simulink model "VINS"  (R2018a)
settings: Solver=FixedStepDiscrete  StartTime=0.0  StopTime=inf  FixedStep=1/Fs  RelTol=1e-3  EnableMultiTasking=on
PreLoadFcn:
  | modelDef = getModelDef(calibrateSFMA);
  | 
  | %imuPar = getImuPar('lmvpUncalibrated');
  | 
  | timeMatchThreshold = 1000;
undefined symbols (not defined in the file or in its folder): beep, dejitter_on, Fs, homogeneous3x4Transform_k_kmin1, imuLocationMm, imuPar, numStates, simData, tstamp_k_us, tstamp_kmin1_us
libraries: simulink x69, dspmtrx3 x35, dspindex x9, vrlib x7, dspstat3 x7, dspinverses x6, dspsigops x5, dspmathops x2, rtwdemowidgets x1, dspfactors x1, simulink_extras x1
(part 1 of 6)
settings Model: SimulationMode=external  TunableVars=dejitter_on,imuLocationMm,imuPar  TunableVarsStorageClass=ExportedGlobal,ExportedGlobal,ExportedGlobal  TunableVarsTypeQualifier=,,const  Creator=Eric  LastModifiedBy=efoxlin
settings SolverCC: PositivePriorityOrder=on
settings DataIOCC: SaveOutput=off  SaveTime=off
settings OptimizationCC: DefaultParameterBehavior=Inlined  UseFloatMulNetSlope=on  DefaultUnderspecifiedDataType=single  UseSpecifiedMinMax=on  PassReuseOutputArgsAs=Individual arguments  NoFixptDivByZeroProtection=on  EfficientFloat2IntCast=on  LifeSpan=1  MaxStackSize=1000000  OptimizeBlockOrder=speed  DifferentSizesBufferReuse=on
settings DebuggingCC: ReadBeforeWriteMsg=DisableAll  WriteAfterWriteMsg=DisableAll  WriteAfterReadMsg=DisableAll  ParameterPrecisionLossMsg=none  ParameterTunabilityLossMsg=error  UnconnectedOutputMsg=none
settings HardwareCC: ProdBitPerPointer=32  ProdBitPerSizeT=32  ProdBitPerPtrDiffT=32  ProdLargestAtomicInteger=Long  ProdLargestAtomicFloat=Double  ProdWordSize=32  ProdHWDeviceType=ARM Compatible->ARM Cortex
settings SFSimCC: MATLABDynamicMemAlloc=off
settings RTWCC: SystemTargetFile=ert.tlc  GenCodeOnly=on  PackageGeneratedCodeAndArtifacts=on  TemplateMakefile=ert_default_tmf  GenerateReport=on  Toolchain=Linaro Toolchain v4.8  BuildConfiguration=Faster Runs  IncludeHyperlinkInReport=on  LaunchReport=on  PortableWordSizes=on  TargetLang=C++  GenerateTraceInfo=on  GenerateTraceReport=on  GenerateTraceReportSl=on  GenerateTraceReportSf=on  GenerateTraceReportEml=on  GenerateCodeReplacementReport=on
settings CodeAppCC: ForceParamTrailComments=on  IgnoreCustomStorageClasses=off  OperatorAnnotations=on  SimulinkDataObjDesc=on  SFDataObjDesc=on  InsertBlockDesc=on
settings ERTTargetCC: TargetLangStandard=C++03 (ISO)  CombineSignalStateStructs=on  SuppressErrorStatus=on  SupportAbsoluteTime=off  MultiInstanceERTCode=on  CodeInterfacePackaging=C++ class  SupportNonFinite=off  SupportComplex=off  SupportVariableSizeSignals=on  RootIOFormat=Structure reference  ERTCustomFileTemplate=example_file_process.tlc  ERTFilePackagingFormat=Compact

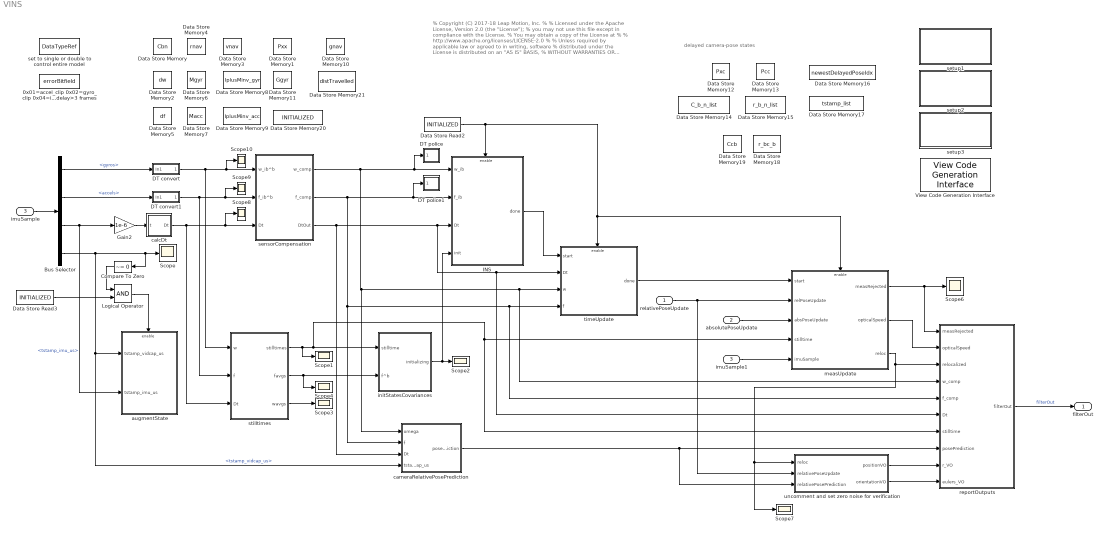
== system VINS ==
  note: delayed camera-pose states
  note: % Copyright (C) 2017-18 Leap Motion, Inc.
      | %
      | %    Licensed under the Apache License, Version 2.0 (the "License");
      | %    you may not use this file except in compliance with the License.
      | %    You may obtain a copy of the License at
      | %
      | %        http://www.apache.org/licenses/LICENSE-2.0
      | %
      | %    Unless required by applicable law or agreed to in writing, software
      | %    distributed under the License is distributed on an "AS IS" BASIS,
      | %    WITHOUT WARRANTIES OR CONDITIONS OF ANY KIND, either express or implied.
      | %    See the License for the specific language governing permissions and
      | %    limitations under the License.
      | % Author: Eric Foxlin
  relativePoseUpdate : Inport  OutDataTypeStr=Bus: relativePoseUpdate
  absolutePoseUpdate : Inport  Port=2  OutDataTypeStr=Bus: absolutePoseUpdate
  imuSample : Inport  Port=3  OutDataTypeStr=Bus: imuSample  PortDimensions=1
  0x01=accel_clip 0x02=gyro_clip 0x04=imu_dropout(>5ms) 0x08=vid_delay>3 frames : DataStoreMemory  DataStoreName=errorBitfield  ReadBeforeWriteMsg=warning  WriteAfterWriteMsg=warning  WriteAfterReadMsg=warning  InitialValue=uint32(0)  ShowAdditionalParam=off  OutDataTypeStr=uint32
  Bus Selector : BusSelector  OutputSignals=gyros,accels,tstamp_imu_us,tstamp_vidcap_us
  Compare To Zero : simulink/Logic and Bit Operations/Compare To Zero  relop=~=  OutDataTypeStr=boolean
  DT convert : Subsystem
  DT convert1 : Subsystem
  DT police : Subsystem  TreatAsAtomicUnit=on
  DT police1 : Subsystem  TreatAsAtomicUnit=on
  Data Store Memory : DataStoreMemory  DataStoreName=Cbn  ReadBeforeWriteMsg=warning  WriteAfterWriteMsg=warning  WriteAfterReadMsg=warning  InitialValue=eye(3)  VectorParams1D=off  ShowAdditionalParam=off
  Data Store Memory1 : DataStoreMemory  DataStoreName=Pxx  ReadBeforeWriteMsg=warning  WriteAfterWriteMsg=warning  WriteAfterReadMsg=warning  InitialValue=eye(modelDef.numStates)*1e-12  ShowAdditionalParam=off
  Data Store Memory10 : DataStoreMemory  DataStoreName=gnav  ReadBeforeWriteMsg=warning  WriteAfterWriteMsg=warning  WriteAfterReadMsg=warning  InitialValue=[0;0; 9.80665]  VectorParams1D=off  ShowAdditionalParam=off
  Data Store Memory11 : DataStoreMemory  DataStoreName=Ggyr  ReadBeforeWriteMsg=warning  WriteAfterWriteMsg=warning  WriteAfterReadMsg=warning  InitialValue=zeros(3,3)  VectorParams1D=off  ShowAdditionalParam=off
  Data Store Memory12 : DataStoreMemory  DataStoreName=Pxc  ReadBeforeWriteMsg=warning  WriteAfterWriteMsg=warning  WriteAfterReadMsg=warning  InitialValue=zeros(modelDef.numStates, modelDef.maxNumDelayedPoses * modelDef.statesPerDelayedPose)  ShowAdditionalParam=off
  Data Store Memory13 : DataStoreMemory  DataStoreName=Pcc  ReadBeforeWriteMsg=warning  WriteAfterWriteMsg=warning  WriteAfterReadMsg=warning  InitialValue=zeros(modelDef.statesPerDelayedPose*modelDef.maxNumDelayedPoses , modelDef.statesPerDelayedPose*modelDef.maxNumDelayedPoses )  ShowAdditionalParam=off
  Data Store Memory14 : DataStoreMemory  DataStoreName=C_b_n_list  ReadBeforeWriteMsg=warning  WriteAfterWriteMsg=warning  WriteAfterReadMsg=warning  InitialValue=zeros(3, 3, max(2,modelDef.maxNumDelayedPoses))  VectorParams1D=off  ShowAdditionalParam=off
  Data Store Memory15 : DataStoreMemory  DataStoreName=r_b_n_list  ReadBeforeWriteMsg=warning  WriteAfterWriteMsg=warning  WriteAfterReadMsg=warning  InitialValue=zeros(3, 1, max(2,modelDef.maxNumDelayedPoses))  VectorParams1D=off  ShowAdditionalParam=off
  Data Store Memory16 : DataStoreMemory  DataStoreName=newestDelayedPoseIdx  ReadBeforeWriteMsg=warning  WriteAfterWriteMsg=warning  WriteAfterReadMsg=warning  ShowAdditionalParam=off  OutDataTypeStr=uint8
  Data Store Memory17 : DataStoreMemory  DataStoreName=tstamp_list  ReadBeforeWriteMsg=warning  WriteAfterWriteMsg=warning  WriteAfterReadMsg=warning  InitialValue=zeros(modelDef.maxNumDelayedPoses, 1)  ShowAdditionalParam=off
  Data Store Memory18 : DataStoreMemory  DataStoreName=r_bc_b  ReadBeforeWriteMsg=warning  WriteAfterWriteMsg=warning  WriteAfterReadMsg=warning  InitialValue=-[-17.48; -4.5; 2.539]/1000  VectorParams1D=off  ShowAdditionalParam=off
  Data Store Memory19 : DataStoreMemory  DataStoreName=Ccb  ReadBeforeWriteMsg=warning  WriteAfterWriteMsg=warning  WriteAfterReadMsg=warning  InitialValue=eye(3)  VectorParams1D=off  ShowAdditionalParam=off
  Data Store Memory2 : DataStoreMemory  DataStoreName=dw  ReadBeforeWriteMsg=warning  WriteAfterWriteMsg=warning  WriteAfterReadMsg=warning  InitialValue=[0;0;0]  VectorParams1D=off  ShowAdditionalParam=off
  Data Store Memory20 : DataStoreMemory  DataStoreName=INITIALIZED  WriteAfterWriteMsg=warning  WriteAfterReadMsg=warning  InitialValue=false  ShowAdditionalParam=off
  Data Store Memory21 : DataStoreMemory  DataStoreName=distTravelled  ReadBeforeWriteMsg=warning  WriteAfterWriteMsg=warning  WriteAfterReadMsg=warning  ShowAdditionalParam=off
  Data Store Memory3 : DataStoreMemory  DataStoreName=vnav  ReadBeforeWriteMsg=warning  WriteAfterWriteMsg=warning  WriteAfterReadMsg=warning  InitialValue=[0;0;0]  VectorParams1D=off  ShowAdditionalParam=off
  Data Store Memory4 : DataStoreMemory  DataStoreName=rnav  ReadBeforeWriteMsg=warning  WriteAfterWriteMsg=warning  WriteAfterReadMsg=warning  InitialValue=[-17.48; -4.5; 2.539]/1000;  VectorParams1D=off  ShowAdditionalParam=off
  Data Store Memory5 : DataStoreMemory  DataStoreName=df  ReadBeforeWriteMsg=warning  WriteAfterWriteMsg=warning  WriteAfterReadMsg=warning  InitialValue=[0;0;0]  VectorParams1D=off  ShowAdditionalParam=off
  Data Store Memory6 : DataStoreMemory  DataStoreName=Mgyr  ReadBeforeWriteMsg=warning  WriteAfterWriteMsg=warning  WriteAfterReadMsg=warning  InitialValue=zeros(3,3)  VectorParams1D=off  ShowAdditionalParam=off
  Data Store Memory7 : DataStoreMemory  DataStoreName=Macc  ReadBeforeWriteMsg=warning  WriteAfterWriteMsg=warning  WriteAfterReadMsg=warning  InitialValue=zeros(3,3)  VectorParams1D=off  ShowAdditionalParam=off
  Data Store Memory8 : DataStoreMemory  DataStoreName=IplusMinv_gyr  WriteAfterWriteMsg=warning  WriteAfterReadMsg=warning  InitialValue=eye(3)  VectorParams1D=off  ShowAdditionalParam=off
  Data Store Memory9 : DataStoreMemory  DataStoreName=IplusMinv_acc  ReadBeforeWriteMsg=warning  WriteAfterWriteMsg=warning  WriteAfterReadMsg=warning  InitialValue=eye(3)  VectorParams1D=off  ShowAdditionalParam=off
  Data Store Read2 : DataStoreRead  Priority=2  DataStoreName=INITIALIZED
  Data Store Read3 : DataStoreRead  DataStoreName=INITIALIZED
  Gain2 : Gain  Gain=1e-6
  INS : Subsystem  Priority=2  TreatAsAtomicUnit=on
      settings: RTWSystemCode=Nonreusable function  RTWFcnNameOpts=Use subsystem name
  Logical Operator : Logic  AllPortsSameDT=off  OutDataTypeStr=boolean
  Scope{,1..4,6..10} (10 alike) : Scope
  View Code Generation Interface : rtwdemowidgets/View Code Generation Interface  SystemSampleTime=-1
      settings: SourceProductName=Simulink Coder  SourceProductBaseCode=RT
  augmentState : Subsystem  Priority=1  TreatAsAtomicUnit=on
      settings: RTWSystemCode=Nonreusable function  RTWFcnNameOpts=Use subsystem name
  calcDt : Subsystem
  cameraRelativePosePrediction : Subsystem  Priority=1  TreatAsAtomicUnit=on
      settings: RTWSystemCode=Nonreusable function  RTWFcnNameOpts=Use subsystem name
  imuSample1 : InportShadow  Port=3  OutDataTypeStr=Bus: imuSample  PortDimensions=1
  initStatesCovariances : Subsystem  Priority=1  TreatAsAtomicUnit=on
      settings: RTWSystemCode=Nonreusable function  RTWFcnNameOpts=Use subsystem name
  measUpdate : Subsystem  TreatAsAtomicUnit=on
      settings: RTWSystemCode=Nonreusable function  RTWFcnNameOpts=Use subsystem name
  reportOutputs : Subsystem  Priority=2  TreatAsAtomicUnit=on
      settings: RTWSystemCode=Nonreusable function  RTWFcnNameOpts=Use subsystem name
  sensorCompensation : Subsystem  TreatAsAtomicUnit=on
      settings: RTWSystemCode=Nonreusable function  RTWFcnNameOpts=Use subsystem name
  set to single or double to control entire model : DataStoreMemory  DataStoreName=DataTypeRef  ReadBeforeWriteMsg=warning  WriteAfterWriteMsg=warning  WriteAfterReadMsg=warning  ShowAdditionalParam=off  OutDataTypeStr=single
  setup1 : Subsystem
      settings: OpenFcn=|
      | set_param(bdroot,'TargetLang','C');
      | set_param(bdroot, 'TargetLangStandard', 'C89/C90 (ANSI)', 'CodeReplacementLibrary','None');
      | dlg = get_param(bdroot, 'SimPrmDialog');
      | if isa(dlg, 'DAStudio.Dialog')
      |             dlg.refresh;
      | end; clear dlg;
      mask Display: disp('Use C89/C90 (ANSI)\nMath Library \n(double-click)')
  setup2 : Subsystem
      settings: OpenFcn=|
      | set_param(bdroot,'TargetLang','C');
      | set_param(bdroot, 'TargetLangStandard', 'C99 (ISO)', 'CodeReplacementLibrary','None');
      | dlg = get_param(bdroot, 'SimPrmDialog');
      | if isa(dlg, 'DAStudio.Dialog')
      |             dlg.refresh;
      | end; clear dlg;
      mask Display: disp('Use C99 (ISO)\nMath Library \n(double-click)')
  setup3 : Subsystem
      settings: OpenFcn=|
      | set_param(bdroot, 'TargetLang', 'C++');
      | set_param(bdroot, 'TargetLangStandard', 'C++03 (ISO)', 'CodeReplacementLibrary','None');
      | set_param(bdroot, 'GenerateCodeMetricsReport','Off'); % not supported with C++
      | dlg = get_param(bdroot, 'SimPrmDialog');
      | if isa(dlg, 'DAStudio.Dialog')
      |             dlg.refresh;
      | end; clear dlg;
      mask Display: disp('Use C++03 (ISO)\nMath Library \n(double-click)')
  stilltimes : Subsystem  TreatAsAtomicUnit=on
      settings: RTWSystemCode=Nonreusable function  RTWFcnNameOpts=Use subsystem name
  timeUpdate : Subsystem  Priority=3  TreatAsAtomicUnit=on
      settings: RTWSystemCode=Nonreusable function  RTWFcnNameOpts=Use subsystem name
  uncomment and set zero noise for verification : Subsystem  TreatAsAtomicUnit=on
  filterOut : Outport  OutDataTypeStr=Bus: filterOut  BusOutputAsStruct=on
  wires:
  sensorCompensation/1(w_comp) -> INS/1(w_ib), DT police/1(In1), cameraRelativePosePrediction/1(omega), timeUpdate/3(w), reportOutputs/4(w_comp)
  INS/1(done) -> timeUpdate/1(start)
  sensorCompensation/3(DtOut) -> cameraRelativePosePrediction/3(Dt), INS/3(Dt), reportOutputs/6(Dt), timeUpdate/2(Dt)
  sensorCompensation/2(f_comp) -> INS/2(f_ib), DT police1/1(In1), cameraRelativePosePrediction/2(f), timeUpdate/4(f), reportOutputs/5(f_comp)
  Bus Selector/2 -> DT convert1/1(In1)  "<accels>"
  Bus Selector/1 -> DT convert/1(In1)  "<gyros>"
  Bus Selector/3 -> augmentState/2(tstamp_imu_us), Gain2/1  "<tstamp_imu_us>"
  initStatesCovariances/1(initializing) -> INS/4(init), Scope2/1
  Data Store Read2/1 -> INS/Enable, measUpdate/Enable, timeUpdate/Enable
  reportOutputs/1(filterOut) -> filterOut/1  "filterOut"
  timeUpdate/1(done) -> measUpdate/1(start)
  stilltimes/2(favgs) -> initStatesCovariances/2(f^b), Scope4/1
  stilltimes/1(stilltimes) -> Scope1/1, reportOutputs/7(stilltime), measUpdate/4(stilltime), initStatesCovariances/1(stilltime)
  stilltimes/3(wavgs) -> Scope3/1
  imuSample/1 -> Bus Selector/1
  calcDt/1(Dt) -> stilltimes/3(Dt), Scope8/1, sensorCompensation/3(Dt)
  Gain2/1 -> calcDt/1(t)
  Bus Selector/4 -> cameraRelativePosePrediction/4(tstamp_vidcap_us), augmentState/1(tstamp_vidcap_us), Compare To Zero/1, Scope/1  "<tstamp_vidcap_us>"
  relativePoseUpdate/1 -> measUpdate/2(relPoseUpdate), uncomment and set zero noise for verification/2(relativePoseUpdate)
  Logical Operator/1 -> augmentState/Enable
  Data Store Read3/1 -> Logical Operator/2
  Compare To Zero/1 -> Logical Operator/1
  imuSample1/1 -> measUpdate/5(imuSample)
  measUpdate/1(measRejected) -> reportOutputs/1(measRejected), Scope6/1
  cameraRelativePosePrediction/1(posePrediction) -> reportOutputs/8(posePrediction), uncomment and set zero noise for verification/3(relativePosePrediction)
  DT convert/1(Out1) -> Scope10/1, sensorCompensation/1(w_ib^b), stilltimes/1(w)
  DT convert1/1(Out1) -> stilltimes/2(f), Scope9/1, sensorCompensation/2(f_ib^b)
  uncomment and set zero noise for verification/1(positionVO) -> reportOutputs/9(r_VO)
  uncomment and set zero noise for verification/2(orientationVO) -> reportOutputs/10(eulers_VO)
  measUpdate/2(opticalSpeed) -> reportOutputs/2(opticalSpeed)
  absolutePoseUpdate/1 -> measUpdate/3(absPoseUpdate)
  measUpdate/3(reloc) -> Scope7/1, uncomment and set zero noise for verification/1(reloc), reportOutputs/3(relocalized)

== system VINS/DT convert ==
  In1 : Inport
  Data Store Read : DataStoreRead  DataStoreName=DataTypeRef
  Data Type Conversion Inherited : simulink/Signal Attributes/Data Type Conversion Inherited  ConvertRealWorld=Real World Value  DoSatur=off
      settings: SourceProductName=Simulink  SourceProductBaseCode=SL
  Out1 : Outport
  wires:
  Data Type Conversion Inherited/1 -> Out1/1
  Data Store Read/1 -> Data Type Conversion Inherited/1
  In1/1 -> Data Type Conversion Inherited/2

== system VINS/DT convert1 ==
  In1 : Inport
  Data Store Read : DataStoreRead  DataStoreName=DataTypeRef
  Data Type Conversion Inherited : simulink/Signal Attributes/Data Type Conversion Inherited  ConvertRealWorld=Real World Value  DoSatur=off
      settings: SourceProductName=Simulink  SourceProductBaseCode=SL
  Out1 : Outport
  wires:
  In1/1 -> Data Type Conversion Inherited/2
  Data Store Read/1 -> Data Type Conversion Inherited/1
  Data Type Conversion Inherited/1 -> Out1/1

== system VINS/DT police ==
  In1 : Inport
  Data Store Read : DataStoreRead  DataStoreName=DataTypeRef
  Data Type Duplicate : DataTypeDuplicate
  wires:
  Data Store Read/1 -> Data Type Duplicate/1
  In1/1 -> Data Type Duplicate/2

== system VINS/DT police1 ==
  In1 : Inport
  Data Store Read : DataStoreRead  DataStoreName=DataTypeRef
  Data Type Duplicate : DataTypeDuplicate
  wires:
  In1/1 -> Data Type Duplicate/2
  Data Store Read/1 -> Data Type Duplicate/1

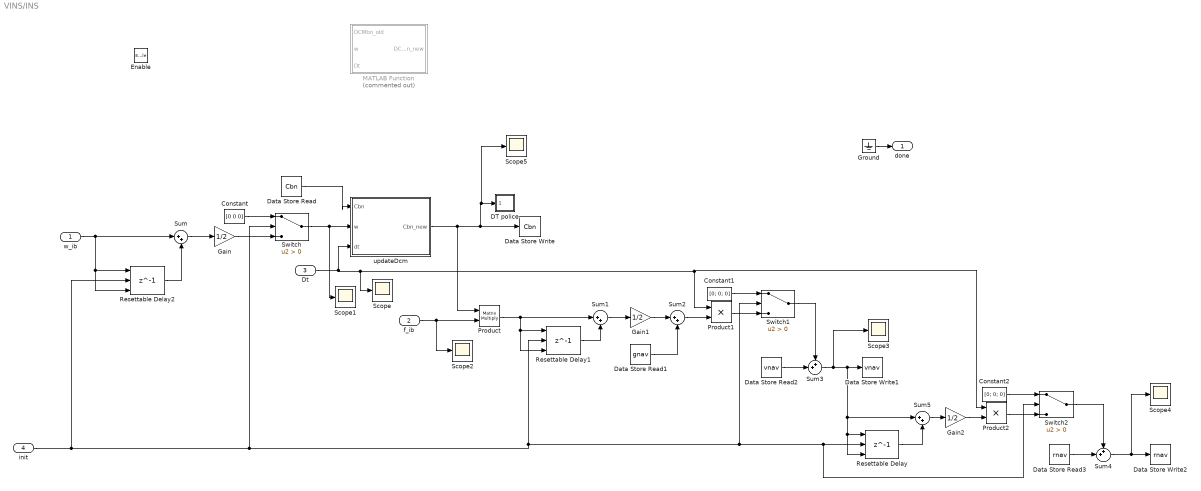
== system VINS/INS ==
  w_ib : Inport
  f_ib : Inport  Port=2
  Dt : Inport  Port=3
  init : Inport  Port=4
  Enable : EnablePort
  Constant : Constant  Value=[0 0 0]
  Constant1 : Constant  Value=[0; 0; 0]  VectorParams1D=off  OutDataTypeStr=Inherit: Inherit via back propagation
  Constant2 : Constant  Value=[0; 0; 0]  VectorParams1D=off  OutDataTypeStr=Inherit: Inherit via back propagation
  DT police : Subsystem  TreatAsAtomicUnit=on
  Data Store Read : DataStoreRead  DataStoreName=Cbn
  Data Store Read1 : DataStoreRead  DataStoreName=gnav
  Data Store Read2 : DataStoreRead  DataStoreName=vnav
  Data Store Read3 : DataStoreRead  DataStoreName=rnav
  Data Store Write : DataStoreWrite  DataStoreName=Cbn
  Data Store Write1 : DataStoreWrite  DataStoreName=vnav
  Data Store Write2 : DataStoreWrite  DataStoreName=rnav
  Gain : Gain  Gain=1/2
  Gain1 : Gain  Gain=1/2
  Gain2 : Gain  Gain=1/2
  Ground : Ground
  MATLAB Function : MATLAB Function  Commented=on  TreatAsAtomicUnit=on
  Product : Product  Multiplication=Matrix(*)
  Product1 : Product
  Product2 : Product
  Resettable Delay : Delay  DelayLength=1  InitialConditionSource=Input port  ExternalReset=Level hold
      settings: InputPortMap=u0,r5,p4
  Resettable Delay1 : Delay  DelayLength=1  InitialConditionSource=Input port  ExternalReset=Level hold
      settings: InputPortMap=u0,r5,p4
  Resettable Delay2 : Delay  DelayLength=1  InitialConditionSource=Input port  ExternalReset=Level hold
      settings: InputPortMap=u0,r5,p4
  Scope{,1..5} (6 alike) : Scope
  Sum{,1..2,5} (4 alike) : Sum  Inputs=|++
  Sum3 : Sum  Inputs=++|
  Sum4 : Sum  Inputs=++|
  Switch : Switch  Criteria=u2 > Threshold
  Switch1 : Switch  Criteria=u2 > Threshold
  Switch2 : Switch  Criteria=u2 > Threshold
  updateDcm : MATLAB Function  TreatAsAtomicUnit=on
  done : Outport
  wires:
  Resettable Delay1/1 -> Sum1/2
  Resettable Delay/1 -> Sum5/2
  Gain2/1 -> Product2/2
  Sum3/1 -> Scope3/1, Data Store Write1/1, Sum5/1, Resettable Delay/1, Resettable Delay/3
  Sum5/1 -> Gain2/1
  Sum4/1 -> Scope4/1, Data Store Write2/1
  Data Store Read3/1 -> Sum4/2
  Switch1/1 -> Sum3/1
  Data Store Read2/1 -> Sum3/2
  Gain1/1 -> Sum2/1
  Sum1/1 -> Gain1/1
  Product/1 -> Sum1/1, Resettable Delay1/1, Resettable Delay1/3
  Sum2/1 -> Product1/2
  Data Store Read1/1 -> Sum2/2
  f_ib/1 -> Scope2/1, Product/2
  Sum/1 -> Gain/1
  Resettable Delay2/1 -> Sum/2
  updateDcm/1(Cbn_new) -> Scope5/1, DT police/1(In1), Data Store Write/1, Product/1
  w_ib/1 -> Sum/1, Resettable Delay2/3, Resettable Delay2/1
  Dt/1 -> updateDcm/3(dt), Scope/1, Product1/1, Product2/1
  init/1 -> Resettable Delay2/2, Switch/2, Switch1/2, Switch2/2, Resettable Delay/2, Resettable Delay1/2
  Data Store Read/1 -> updateDcm/1(Cbn)
  Gain/1 -> Switch/3
  Constant/1 -> Switch/1
  Product1/1 -> Switch1/3
  Constant1/1 -> Switch1/1
  Product2/1 -> Switch2/3
  Switch2/1 -> Sum4/1
  Constant2/1 -> Switch2/1
  Switch/1 -> updateDcm/2(w), Scope1/1
  Ground/1 -> done/1

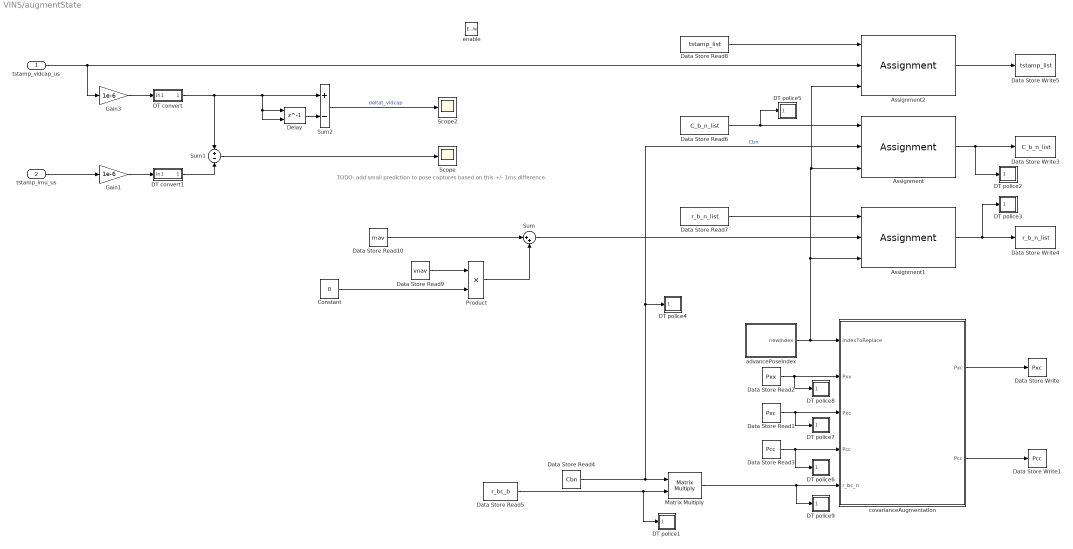
== system VINS/augmentState ==
  note: TODO: add small prediction to pose captures based on this +/- 1ms difference.
  tstamp_vidcap_us : Inport
  tstamp_imu_us : Inport  Port=2
  "enable " : EnablePort
  Assignment : Assignment  NumberOfDimensions=3  DiagnosticForDimensions=Warning  IndexOptions=Index vector (dialog),Index vector (dialog),Index vector (port)  Indices=1:3,1:3,1  OutputSizes=1,1,1
  Assignment1 : Assignment  NumberOfDimensions=3  DiagnosticForDimensions=Warning  IndexOptions=Index vector (dialog),Index vector (dialog),Index vector (port)  Indices=1:3,1,1  OutputSizes=1,1,1
  Assignment2 : Assignment  DiagnosticForDimensions=Warning  IndexOptions=Index vector (port)  Indices=1:3  OutputSizes=1
  Constant : Constant  Value=0  OutDataTypeStr=Inherit: Inherit via back propagation
  DT convert : Subsystem
  DT convert1 : Subsystem
  DT police1 : Subsystem  TreatAsAtomicUnit=on
  DT police2 : Subsystem  TreatAsAtomicUnit=on
  DT police3 : Subsystem  TreatAsAtomicUnit=on
  DT police4 : Subsystem  TreatAsAtomicUnit=on
  DT police5 : Subsystem  TreatAsAtomicUnit=on
  DT police6 : Subsystem  TreatAsAtomicUnit=on
  DT police7 : Subsystem  TreatAsAtomicUnit=on
  DT police8 : Subsystem  TreatAsAtomicUnit=on
  DT police9 : Subsystem  TreatAsAtomicUnit=on
  Data Store Read1 : DataStoreRead  DataStoreName=Pxc
  Data Store Read10 : DataStoreRead  DataStoreName=rnav
  Data Store Read2 : DataStoreRead  DataStoreName=Pxx
  Data Store Read3 : DataStoreRead  DataStoreName=Pcc
  Data Store Read4 : DataStoreRead  DataStoreName=Cbn
  Data Store Read5 : DataStoreRead  DataStoreName=r_bc_b
  Data Store Read6 : DataStoreRead  DataStoreName=C_b_n_list
  Data Store Read7 : DataStoreRead  DataStoreName=r_b_n_list
  Data Store Read8 : DataStoreRead  DataStoreName=tstamp_list
  Data Store Read9 : DataStoreRead  DataStoreName=vnav
  Data Store Write : DataStoreWrite  DataStoreName=Pxc
  Data Store Write1 : DataStoreWrite  DataStoreName=Pcc
  Data Store Write3 : DataStoreWrite  DataStoreName=C_b_n_list
  Data Store Write4 : DataStoreWrite  DataStoreName=r_b_n_list
  Data Store Write5 : DataStoreWrite  DataStoreName=tstamp_list
  Delay : Delay  DelayLength=1  InitialConditionSource=Input port
      settings: InputPortMap=u0,p4
  Gain1 : Gain  Gain=1e-6
  Gain3 : Gain  Gain=1e-6
  Matrix Multiply : Product  Multiplication=Matrix(*)
  Product : Product
  Scope : Scope
  Scope2 : Scope
  Sum : Sum  Inputs=|++
  Sum1 : Sum  Inputs=+-
  Sum2 : Sum  Inputs=+-
  advancePoseIndex : Subsystem
  covarianceAugmentation : MATLAB Function  TreatAsAtomicUnit=on
  wires:
  Data Store Read2/1 -> DT police8/1(In1), covarianceAugmentation/2(Pxx)
  Data Store Read1/1 -> DT police7/1(In1), covarianceAugmentation/3("Pxc ")
  Data Store Read3/1 -> covarianceAugmentation/4("Pcc "), DT police6/1(In1)
  covarianceAugmentation/1(Pxc) -> Data Store Write/1
  covarianceAugmentation/2(Pcc) -> Data Store Write1/1
  Matrix Multiply/1 -> DT police9/1(In1), covarianceAugmentation/5(r_bc_n)
  Data Store Read5/1 -> DT police1/1(In1), Matrix Multiply/2
  Data Store Read6/1 -> DT police5/1(In1), Assignment/1
  Data Store Read7/1 -> Assignment1/1
  Assignment/1 -> DT police2/1(In1), Data Store Write3/1
  Assignment1/1 -> DT police3/1(In1), Data Store Write4/1
  Data Store Read8/1 -> Assignment2/1
  tstamp_vidcap_us/1 -> Gain3/1, Assignment2/2
  Assignment2/1 -> Data Store Write5/1
  Data Store Read4/1 -> Assignment/2, DT police4/1(In1), Matrix Multiply/1  "Cbn"
  Sum/1 -> Assignment1/2
  tstamp_imu_us/1 -> Gain1/1
  Sum1/1 -> Scope/1
  advancePoseIndex/1(newIndex) -> Assignment1/3, Assignment2/3, Assignment/3, covarianceAugmentation/1(indexToReplace)
  Data Store Read10/1 -> Sum/1
  Product/1 -> Sum/2
  Data Store Read9/1 -> Product/1
  Constant/1 -> Product/2
  Gain3/1 -> DT convert/1(In1)
  Sum2/1 -> Scope2/1  "deltat_vidcap"
  DT convert/1(Out1) -> Sum1/1, Delay/2, Delay/1, Sum2/1
  Delay/1 -> Sum2/2
  Gain1/1 -> DT convert1/1(In1)
  DT convert1/1(Out1) -> Sum1/2

== system VINS/calcDt ==
  t : Inport
  Constant : Constant  Value=0
  Constant10 : Constant
  DT convert : Subsystem
  Difference : simulink/Discrete/Difference  ICPrevInput=0.0  OutMin=[]  OutMax=[]  OutDataType=fixdt(1, 16)  OutScaling=2^-10  DoSatur=off
  Switch : Switch  Criteria=u2 > Threshold
  Unit Delay : UnitDelay  SampleTime=-1
  Dt : Outport
  wires:
  Unit Delay/1 -> Switch/2
  Constant/1 -> Switch/3
  Switch/1 -> DT convert/1(In1)
  Difference/1 -> Switch/1
  Constant10/1 -> Unit Delay/1
  t/1 -> Difference/1
  DT convert/1(Out1) -> Dt/1

== system VINS/cameraRelativePosePrediction ==
  omega : Inport
  f : Inport  Port=2
  Dt : Inport  Port=3
  tstamp_vidcap_us : Inport  Port=4
  Compare To Zero : simulink/Logic and Bit Operations/Compare To Zero  relop=~=  OutDataTypeStr=boolean
  Scope : Scope
  Scope1 : Scope
  b frame to c frame : Subsystem  TreatAsAtomicUnit=on
  b frame to c frame1 : Subsystem  TreatAsAtomicUnit=on
  frameToFramePrediction : Subsystem  TreatAsAtomicUnit=on
  localIns : Subsystem  Priority=2  TreatAsAtomicUnit=on
      settings: RTWSystemCode=Nonreusable function  RTWFcnNameOpts=Use subsystem name
  posePrediction : Outport
  wires:
  tstamp_vidcap_us/1 -> frameToFramePrediction/5(tstamp_vidcap_us), Compare To Zero/1
  omega/1 -> localIns/1(w_ib)
  f/1 -> localIns/2(f_ib)
  Dt/1 -> localIns/3(Dt)
  frameToFramePrediction/1(cameraRelativePosePrediction) -> posePrediction/1
  Compare To Zero/1 -> b frame to c frame1/Enable, frameToFramePrediction/Enable, b frame to c frame/Enable, localIns/4(cloneStates)
  localIns/1(Cbn_k) -> Scope1/1, b frame to c frame/1(Cbn)
  localIns/2(rbn_k) -> Scope/1, b frame to c frame/2(r_nb_n)
  b frame to c frame/1(Ccn) -> frameToFramePrediction/1(Ccn_k)
  b frame to c frame/2(rcn) -> frameToFramePrediction/2(r_nc_n_k)
  localIns/3(Cbn_kmin1) -> b frame to c frame1/1(Cbn)
  localIns/4(rbn_kmin1) -> b frame to c frame1/2(r_nb_n)
  b frame to c frame1/1(Ccn) -> frameToFramePrediction/3(Ccn_kmin1)
  b frame to c frame1/2(rcn) -> frameToFramePrediction/4(r_nc_n_kmin1)

== system VINS/initStatesCovariances ==
  stilltime : Inport
  f^b : Inport  Port=2
  Compare To Constant : simulink/Logic and Bit Operations/Compare To Constant  relop=>  const=0.25  OutDataTypeStr=boolean
  Constant : Constant  Value=true
  Constant1 : Constant  Value=false
  Constant2 : Constant  Value=simData
  Constant3 : Constant  Value=false
  DT police : Subsystem  TreatAsAtomicUnit=on
  Data Store Read : DataStoreRead  DataStoreName=INITIALIZED
  Environment Controller : simulink/Signal Routing/Environment Controller
      settings: SourceProductName=Simulink  SourceProductBaseCode=SL
  Environment Controller1 : simulink/Signal Routing/Environment Controller
      settings: SourceProductName=Simulink  SourceProductBaseCode=SL
  Logical Operator : Logic  AllPortsSameDT=off  OutDataTypeStr=boolean
  Logical Operator1 : Logic  Operator=NOT  Inputs=1  IconShape=distinctive  AllPortsSameDT=off  OutDataTypeStr=boolean
  Logical Operator2 : Logic  AllPortsSameDT=off  OutDataTypeStr=boolean
  Logical Operator3 : Logic  AllPortsSameDT=off  OutDataTypeStr=boolean
  Logical Operator4 : Logic  Inputs=3  AllPortsSameDT=off  OutDataTypeStr=boolean
  Logical Operator5 : Logic  Operator=NOT  Inputs=1  IconShape=distinctive  AllPortsSameDT=off  OutDataTypeStr=boolean
  Scope : Scope
  Scope1 : Scope
  Selector : Selector  InputPortWidth=2  IndexOptions=Index vector (dialog)  Indices=2  OutputSizes=1
  Switch : Switch  Criteria=u2 > Threshold
  Unit Delay : UnitDelay  InitialCondition=true  SampleTime=-1
  initialize r_bc_b : Subsystem  TreatAsAtomicUnit=on
  pefectInit (only for development testing) : Subsystem  TreatAsAtomicUnit=on
  realInit : Subsystem
      settings: RTWSystemCode=Nonreusable function  RTWFcnNameOpts=Use subsystem name
  setInitializedFlag : Subsystem
  setP : Subsystem
  use perfect init : Constant  Value=true
  initializing : Outport  OutDataTypeStr=boolean
  wires:
  setP/1(Out1) -> setInitializedFlag/Enable
  setInitializedFlag/1(Out1) -> initializing/1
  Logical Operator1/1 -> Logical Operator/1
  Data Store Read/1 -> Logical Operator1/1
  stilltime/1 -> Selector/1
  Compare To Constant/1 -> Logical Operator/2
  Selector/1 -> Compare To Constant/1
  Environment Controller/1 -> setP/Enable
  Switch/1 -> Environment Controller/1
  pefectInit (only for development testing)/1(Out1) -> Switch/1
  realInit/1(Out1) -> Environment Controller/2, Switch/3
  f^b/1 -> DT police/1(In1), realInit/1(f_ib_b)
  Logical Operator/1 -> Logical Operator3/2, Logical Operator2/1
  Logical Operator2/1 -> Scope/1, setP/1(perfectInit), pefectInit (only for development testing)/Enable
  Logical Operator3/1 -> Scope1/1, realInit/Enable
  Environment Controller1/1 -> Logical Operator4/2
  Constant/1 -> Environment Controller1/1
  Constant1/1 -> Environment Controller1/2
  use perfect init/1 -> Logical Operator4/1
  Logical Operator5/1 -> Logical Operator3/1
  Logical Operator4/1 -> Logical Operator2/2, Switch/2, Logical Operator5/1  "usePerfectInit"
  Constant2/1 -> Logical Operator4/3
  Constant3/1 -> Unit Delay/1
  Unit Delay/1 -> initialize r_bc_b/Enable

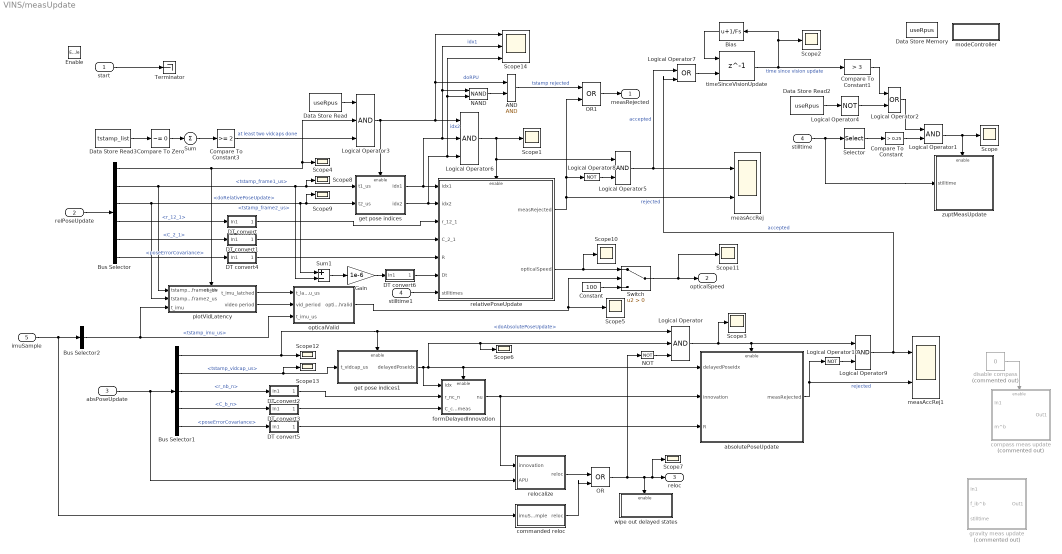
== system VINS/measUpdate ==
  start : Inport
  relPoseUpdate : Inport  Port=2
  absPoseUpdate : Inport  Port=3
  stilltime : Inport  Port=4
  imuSample : Inport  Port=5
  Enable : EnablePort  StatesWhenEnabling=reset  ShowOutputPort=on
  AND : Logic  IconShape=distinctive  AllPortsSameDT=off  OutDataTypeStr=boolean
  Bias : Bias  Bias=1/Fs
  Bus Selector : BusSelector  OutputSignals=doRelativePoseUpdate,tstamp_frame1_us,tstamp_frame2_us,r_12_1,C_2_1,poseErrorCovariance
  Bus Selector1 : BusSelector  OutputSignals=doAbsolutePoseUpdate,tstamp_vidcap_us,r_nb_n,C_b_n,poseErrorCovariance
  Bus Selector2 : BusSelector  OutputSignals=tstamp_imu_us
  Compare To Constant : simulink/Logic and Bit Operations/Compare To Constant  relop=>  const=0.25  OutDataTypeStr=boolean
  Compare To Constant1 : simulink/Logic and Bit Operations/Compare To Constant  relop=>  const=3  OutDataTypeStr=boolean
  Compare To Constant3 : simulink/Logic and Bit Operations/Compare To Constant  relop=>=  const=2  OutDataTypeStr=boolean
  Compare To Zero : simulink/Logic and Bit Operations/Compare To Zero  relop=~=  OutDataTypeStr=boolean
  Constant : Constant  Value=100  OutDataTypeStr=Inherit: Inherit via back propagation
  DT convert : Subsystem
  DT convert1 : Subsystem
  DT convert2 : Subsystem
  DT convert3 : Subsystem
  DT convert4 : Subsystem
  DT convert5 : Subsystem
  DT convert6 : Subsystem
  Data Store Memory : DataStoreMemory  DataStoreName=useRpus  ReadBeforeWriteMsg=warning  WriteAfterWriteMsg=warning  WriteAfterReadMsg=warning  InitialValue=true  ShowAdditionalParam=off
  Data Store Read : DataStoreRead  DataStoreName=useRpus
  Data Store Read2 : DataStoreRead  DataStoreName=useRpus
  Data Store Read3 : DataStoreRead  DataStoreName=tstamp_list
  Gain : Gain  Gain=1e-6
  Logical Operator : Logic  Inputs=3  AllPortsSameDT=off  OutDataTypeStr=boolean
  Logical Operator1 : Logic  AllPortsSameDT=off  OutDataTypeStr=boolean
  Logical Operator10 : Logic  Operator=NOT  IconShape=distinctive  AllPortsSameDT=off  OutDataTypeStr=boolean
  Logical Operator2 : Logic  Operator=OR  AllPortsSameDT=off  OutDataTypeStr=boolean
  Logical Operator3 : Logic  Inputs=3  AllPortsSameDT=off  OutDataTypeStr=boolean
  Logical Operator4 : Logic  Operator=NOT  IconShape=distinctive  AllPortsSameDT=off  OutDataTypeStr=boolean
  Logical Operator5 : Logic  AllPortsSameDT=off  OutDataTypeStr=boolean
  Logical Operator6 : Logic  Inputs=3  AllPortsSameDT=off  OutDataTypeStr=boolean
  Logical Operator7 : Logic  Operator=OR  IconShape=distinctive  AllPortsSameDT=off  OutDataTypeStr=boolean
  Logical Operator8 : Logic  Operator=NOT  IconShape=distinctive  AllPortsSameDT=off  OutDataTypeStr=boolean
  Logical Operator9 : Logic  AllPortsSameDT=off  OutDataTypeStr=boolean
  NAND : Logic  Operator=NAND  IconShape=distinctive  AllPortsSameDT=off  OutDataTypeStr=boolean
  NOT : Logic  Operator=NOT  IconShape=distinctive  AllPortsSameDT=off  OutDataTypeStr=boolean
  OR : Logic  Operator=OR  IconShape=distinctive  AllPortsSameDT=off  OutDataTypeStr=boolean
  OR1 : Logic  Operator=OR  IconShape=distinctive  AllPortsSameDT=off  OutDataTypeStr=boolean
  Scope{,1..13} (14 alike) : Scope
  Scope14 : Scope  NumInputPorts=3
  Selector : Selector  InputPortWidth=2  IndexOptions=Index vector (dialog)  Indices=2  OutputSizes=1
  Sum : Sum  Inputs=+
  Sum1 : Sum  Inputs=+-
  Switch : Switch  Criteria=u2 > Threshold
  Terminator : Terminator
  absolutePoseUpdate : Subsystem  Priority=4  TreatAsAtomicUnit=on
      settings: RTWSystemCode=Nonreusable function  RTWFcnNameOpts=Use subsystem name
  commanded reloc : Subsystem
  compass meas update : Subsystem  Commented=on  TreatAsAtomicUnit=on
  disable compass : Constant  Commented=on  Value=0
  formDelayedInnovation : Subsystem  TreatAsAtomicUnit=on
  get pose indices : Subsystem  TreatAsAtomicUnit=on
  get pose indices1 : Subsystem  TreatAsAtomicUnit=on
  gravity meas update : Subsystem  Commented=on  TreatAsAtomicUnit=on
  measAccRej : Scope  NumInputPorts=2
  measAccRej1 : Scope  NumInputPorts=2
  modeController : Subsystem
  opticalValid : Subsystem  TreatAsAtomicUnit=on
  plotVidLatency : Subsystem
  relativePoseUpdate : Subsystem  Priority=4  TreatAsAtomicUnit=on
      settings: RTWSystemCode=Nonreusable function  RTWFcnNameOpts=Use subsystem name
  relocalize : Subsystem  TreatAsAtomicUnit=on
  stilltime1 : InportShadow  Port=4
  timeSinceVisionUpdate : Delay  DelayLength=1  InitialCondition=0  ExternalReset=Level
      settings: InputPortMap=u0,r5
  wipe out delayed states : Subsystem  TreatAsAtomicUnit=on
  zuptMeasUpdate : Subsystem  Priority=4  TreatAsAtomicUnit=on
      settings: RTWSystemCode=Nonreusable function  RTWFcnNameOpts=Use subsystem name
  measRejected : Outport
  opticalSpeed : Outport  Port=2  InitialOutput=100
  reloc : Outport  Port=3  OutputWhenDisabled=reset  InitialOutput=false
  wires:
  Logical Operator1/1 -> Scope/1, zuptMeasUpdate/Enable
  stilltime/1 -> Selector/1, zuptMeasUpdate/1(stilltime)
  start/1 -> Terminator/1
  Selector/1 -> Compare To Constant/1
  disable compass/1 -> compass meas update/Enable
  relPoseUpdate/1 -> Bus Selector/1
  Bus Selector/1 -> Scope4/1, Logical Operator3/2, plotVidLatency/Enable  "<doRelativePoseUpdate>"
  Bus Selector/2 -> get pose indices/1(t1_us), Scope8/1, Sum1/2, plotVidLatency/1(tstamp_frame1_us)  "<tstamp_frame1_us>"
  Bus Selector/3 -> get pose indices/2(t2_us), Scope9/1, Sum1/1, plotVidLatency/2(tstamp_frame2_us)  "<tstamp_frame2_us>"
  Bus Selector/4 -> DT convert/1(In1)  "<r_12_1>"
  Bus Selector/5 -> DT convert1/1(In1)  "<C_2_1>"
  Bias/1 -> timeSinceVisionUpdate/1
  timeSinceVisionUpdate/1 -> Compare To Constant1/1, Scope2/1, Bias/1  "time since vision update"
  Compare To Constant/1 -> Logical Operator1/2
  Logical Operator2/1 -> Logical Operator1/1
  Compare To Constant1/1 -> Logical Operator2/1
  Logical Operator3/1 -> AND/1, Scope14/1, Logical Operator6/1, get pose indices/Enable  "doRPU"
  Data Store Read/1 -> Logical Operator3/1
  Logical Operator4/1 -> Logical Operator2/2
  Data Store Read2/1 -> Logical Operator4/1
  Data Store Read3/1 -> Compare To Zero/1
  Compare To Constant3/1 -> Logical Operator3/3  "at least two vidcaps done"
  get pose indices/1(idx1) -> Scope14/2, NAND/1, Logical Operator6/2, relativePoseUpdate/1(idx1)  "idx1"
  get pose indices/2(idx2) -> Scope14/3, NAND/2, Logical Operator6/3, relativePoseUpdate/2(idx2)  "idx2"
  Logical Operator6/1 -> Scope1/1, relativePoseUpdate/Enable, Logical Operator5/1
  absPoseUpdate/1 -> relocalize/2(APU), Bus Selector1/1
  Bus Selector1/3 -> DT convert2/1(In1)  "<r_nb_n>"
  Bus Selector1/4 -> DT convert3/1(In1)  "<C_b_n>"
  Bus Selector1/1 -> Scope12/1, get pose indices1/Enable, Logical Operator/1  "<doAbsolutePoseUpdate>"
  get pose indices1/1(delayedPoseIdx) -> formDelayedInnovation/1(idx), Scope6/1, Logical Operator/2, formDelayedInnovation/Enable, absolutePoseUpdate/1(delayedPoseIdx)
  Bus Selector1/2 -> Scope13/1, get pose indices1/1(t_vidcap_us)  "<tstamp_vidcap_us>"
  Bus Selector2/1 -> opticalValid/3(t_imu_us), plotVidLatency/3(t_imu)  "<tstamp_imu_us>"
  Logical Operator7/1 -> timeSinceVisionUpdate/2
  Compare To Zero/1 -> Sum/1
  Sum/1 -> Compare To Constant3/1
  DT convert1/1(Out1) -> relativePoseUpdate/4(C_2_1)
  Bus Selector/6 -> DT convert4/1(In1)  "<poseErrorCovariance>"
  DT convert4/1(Out1) -> relativePoseUpdate/5(R)
  Bus Selector1/5 -> DT convert5/1(In1)  "<poseErrorCovariance>"
  DT convert5/1(Out1) -> absolutePoseUpdate/3(R)
  relativePoseUpdate/1(measRejected) -> measAccRej/2, OR1/2, Logical Operator8/1  "rejected"
  Logical Operator8/1 -> Logical Operator5/2
  Logical Operator5/1 -> measAccRej/1, Logical Operator7/1  "accepted"
  DT convert/1(Out1) -> relativePoseUpdate/3(r_12_1)
  Sum1/1 -> Gain/1
  Gain/1 -> DT convert6/1(In1)
  stilltime1/1 -> relativePoseUpdate/7(stilltimes)
  relativePoseUpdate/2(opticalSpeed) -> Scope10/1, Switch/1
  DT convert6/1(Out1) -> relativePoseUpdate/6(Dt)
  plotVidLatency/1(t_imu_latched) -> opticalValid/1(t_lastRpu_us)
  plotVidLatency/2(video period) -> opticalValid/2(vid_period)
  opticalValid/1("opticalValid ") -> Scope5/1, Switch/2
  Switch/1 -> Scope11/1, opticalSpeed/1
  Constant/1 -> Switch/3
  formDelayedInnovation/1(nu) -> absolutePoseUpdate/2(innovation), relocalize/1(innovation)
  DT convert2/1(Out1) -> formDelayedInnovation/2(r_nc_n)
  DT convert3/1(Out1) -> formDelayedInnovation/3(C_c_n_meas)
  relocalize/1(reloc) -> OR/1
  NOT/1 -> Logical Operator/3
  imuSample/1 -> commanded reloc/1(imuSample), Bus Selector2/1
  commanded reloc/1(reloc) -> OR/2
  OR/1 -> Scope7/1, reloc/1, wipe out delayed states/Enable, NOT/1
  Logical Operator10/1 -> Logical Operator9/2
  absolutePoseUpdate/1(measRejected) -> Logical Operator10/1, measAccRej1/2  "rejected"
  Logical Operator/1 -> Logical Operator9/1, absolutePoseUpdate/Enable, Scope3/1
  Logical Operator9/1 -> Logical Operator7/2, measAccRej1/1  "accepted"
  NAND/1 -> AND/2
  OR1/1 -> measRejected/1
  AND/1 -> OR1/1  "tstamp rejected"

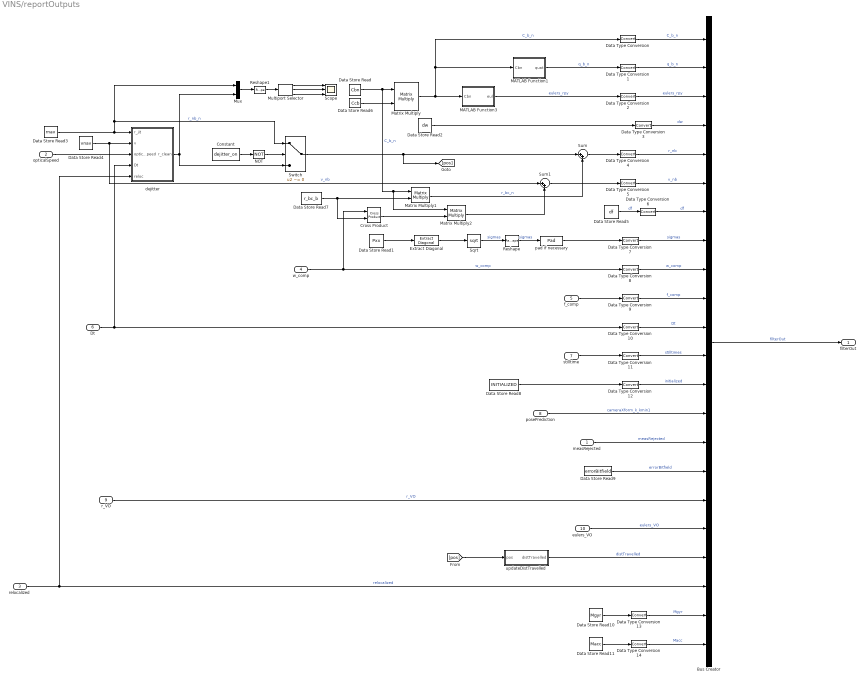
== system VINS/reportOutputs ==
  measRejected : Inport
  opticalSpeed : Inport  Port=2
  relocalized : Inport  Port=3
  w_comp : Inport  Port=4
  f_comp : Inport  Port=5
  Dt : Inport  Port=6
  stilltime : Inport  Port=7
  posePrediction : Inport  Port=8
  r_VO : Inport  Port=9
  eulers_VO : Inport  Port=10
  Bus Creator : BusCreator  Inputs=22  OutDataTypeStr=Bus: filterOut  NonVirtualBus=on
  Constant : Constant  Value=dejitter_on
  Cross Product : vrlib/Utilities/Cross Product
      settings: SourceProductBaseCode=VR
  Data Store Read : DataStoreRead  DataStoreName=Cbn
  Data Store Read1 : DataStoreRead  DataStoreName=Pxx
  Data Store Read10 : DataStoreRead  DataStoreName=Mgyr
  Data Store Read11 : DataStoreRead  DataStoreName=Macc
  Data Store Read2 : DataStoreRead  DataStoreName=dw
  Data Store Read3 : DataStoreRead  DataStoreName=rnav
  Data Store Read4 : DataStoreRead  DataStoreName=vnav
  Data Store Read5 : DataStoreRead  DataStoreName=df
  Data Store Read6 : DataStoreRead  DataStoreName=Ccb
  Data Store Read7 : DataStoreRead  DataStoreName=r_bc_b
  Data Store Read8 : DataStoreRead  Priority=2  DataStoreName=INITIALIZED
  Data Store Read9 : DataStoreRead  DataStoreName=errorBitfield
  Data Type Conversion{,1..14} (15 alike) : DataTypeConversion
  Extract Diagonal : dspmtrx3/Extract Diagonal
      settings: SourceProductName=DSP System Toolbox  SourceProductBaseCode=DS
  MATLAB Function1 : MATLAB Function  TreatAsAtomicUnit=on
  MATLAB Function3 : MATLAB Function  TreatAsAtomicUnit=on
  Matrix Multiply : Product  Multiplication=Matrix(*)
  Matrix Multiply1 : Product  Multiplication=Matrix(*)
  Matrix Multiply2 : Product  Multiplication=Matrix(*)
  Multiport Selector : dspindex/Multiport Selector  rowsOrCols=Rows  idxCellArray={1,2,3 }  idxErrMode=Clip Index
  Mux : Mux  Inputs=2
  NOT : Logic  Operator=NOT  IconShape=distinctive  AllPortsSameDT=off  OutDataTypeStr=boolean
  Reshape : Reshape  OutputDimensionality=Column vector (2-D)
  Reshape1 : Reshape  OutputDimensionality=Customize  OutputDimensions=[3,2]
  Scope : Scope  NumInputPorts=3
  Sqrt : Sqrt  SaturateOnIntegerOverflow=on
  Sum : Sum  Inputs=|++
  Sum1 : Sum  Inputs=|++
  Switch : Switch  Criteria=u2 ~= 0
  dejitter : Subsystem  TreatAsAtomicUnit=on
  pad if necessary : dspsigops/Pad  padAlong=Columns  dimsToPad=1  valSrc=Specify via dialog  padVal=0  spec=Output size  padNumOutRowsSpecMethod=User-specified  numOutRows=33  padNumOutColsSpecMethod=User-specified  numOutCols=1  isVarDimsMode=off  padBeginning=0  padEnd=0  outSizeMode=User-specified  outSize=1  padSigAt=End  trunc_flag=None  roundingMode=Floor  overflowMode=off  truncOrWrapMode=Truncate  wrap_flag=None
      settings: SourceProductName=DSP System Toolbox  SourceProductBaseCode=DS
  updateDistTravelled : Subsystem  TreatAsAtomicUnit=on
  filterOut : Outport  OutDataTypeStr=Bus: filterOut
  wires:
  Reshape/1 -> pad if necessary/1  "sigmas"
  stilltime/1 -> Data Type Conversion11/1
  Dt/1 -> Data Type Conversion10/1, dejitter/4(Dt)
  MATLAB Function1/1(quat) -> Data Type Conversion1/1  "q_b_n"
  MATLAB Function3/1(eul) -> Data Type Conversion2/1  "eulers_rpy"
  Sum/1 -> Data Type Conversion4/1
  Data Store Read2/1 -> Data Type Conversion3/1
  Sum1/1 -> Data Type Conversion5/1
  w_comp/1 -> Data Type Conversion8/1, Cross Product/1  "w_comp"
  Data Store Read5/1 -> Data Type Conversion6/1  "df"
  f_comp/1 -> Data Type Conversion9/1
  Sqrt/1 -> Reshape/1  "sigmas"
  Bus Creator/1 -> filterOut/1  "filterOut"
  Data Store Read1/1 -> Extract Diagonal/1
  Extract Diagonal/1 -> Sqrt/1
  Matrix Multiply/1 -> MATLAB Function3/1(Cbn), Data Type Conversion/1, MATLAB Function1/1(Cbn)  "C_b_n"
  pad if necessary/1 -> Data Type Conversion7/1
  Data Store Read8/1 -> Data Type Conversion12/1
  Data Store Read6/1 -> Matrix Multiply/2
  Data Store Read/1 -> Matrix Multiply2/1, Matrix Multiply1/1, Matrix Multiply/1  "C_b_n"
  Data Store Read7/1 -> Cross Product/2, Matrix Multiply1/2
  Data Store Read3/1 -> Switch/1, Mux/1, dejitter/1(r_jit)  "r_nb_n"
  Matrix Multiply1/1 -> Sum/2  "r_bc_n"
  Data Store Read4/1 -> Sum1/1, dejitter/2(v)  "v_nb"
  Matrix Multiply2/1 -> Sum1/2
  Cross Product/1 -> Matrix Multiply2/2
  Data Type Conversion/1 -> Bus Creator/1  "C_b_n"
  Data Type Conversion1/1 -> Bus Creator/2  "q_b_n"
  Data Type Conversion2/1 -> Bus Creator/3  "eulers_rpy"
  Data Type Conversion3/1 -> Bus Creator/4  "dw"
  Data Type Conversion4/1 -> Bus Creator/5  "r_nb"
  Data Type Conversion5/1 -> Bus Creator/6  "v_nb"
  Data Type Conversion6/1 -> Bus Creator/7  "df"
  Data Type Conversion7/1 -> Bus Creator/8  "sigmas"
  Data Type Conversion8/1 -> Bus Creator/9  "w_comp"
  Data Type Conversion9/1 -> Bus Creator/10  "f_comp"
  Data Type Conversion10/1 -> Bus Creator/11  "Dt"
  Data Type Conversion11/1 -> Bus Creator/12  "stilltimes"
  Data Type Conversion12/1 -> Bus Creator/13  "initialized"
  posePrediction/1 -> Bus Creator/14  "cameraXform_k_kmin1"
  measRejected/1 -> Bus Creator/15  "measRejected"
  Switch/1 -> [pos], Sum/1
  Mux/1 -> Reshape1/1
  Reshape1/1 -> Multiport Selector/1
  Multiport Selector/1 -> Scope/1
  Multiport Selector/2 -> Scope/2
  Multiport Selector/3 -> Scope/3
  Data Store Read9/1 -> Bus Creator/16  "errorBitfield"
  r_VO/1 -> Bus Creator/17  "r_VO"
  eulers_VO/1 -> Bus Creator/18  "eulers_VO"
  [pos] -> updateDistTravelled/1(pos)
  updateDistTravelled/1(distTravelled) -> Bus Creator/19  "distTravelled"
  Data Store Read10/1 -> Data Type Conversion13/1
  Data Store Read11/1 -> Data Type Conversion14/1
  Data Type Conversion13/1 -> Bus Creator/21  "Mgyr"
  Data Type Conversion14/1 -> Bus Creator/22  "Macc"
  opticalSpeed/1 -> dejitter/3(opticalSpeed)
  dejitter/1(r_clean) -> Switch/3, Mux/2
  relocalized/1 -> dejitter/5(reloc), Bus Creator/20  "relocalized"
  Constant/1 -> NOT/1
  NOT/1 -> Switch/2

== system VINS/sensorCompensation ==
  note: w_meas = w_true + dw + Mgyr * w_true + Ggyr * f_true
      | w_comp = (I + Mgyr) -1 * (w_meas - dw - Ggyr * f_true)
      |
      | f_meas = f_true + df + Macc * f_true
      | f_comp = (I + Macc) -1 * (f_meas - df)
  w_ib^b : Inport  Unit=rad/s
  f_ib^b : Inport  Port=2  Unit=m/s^2  PortDimensions=3
  Dt : Inport  Port=3  Unit=rad/s
  Compare To Constant : simulink/Logic and Bit Operations/Compare To Constant  relop=>  const=0.005  OutDataTypeStr=boolean
  Compare To Constant1 : simulink/Logic and Bit Operations/Compare To Constant  relop=<  const=0  OutDataTypeStr=boolean
  DT police : Subsystem  TreatAsAtomicUnit=on
  DT police1 : Subsystem  TreatAsAtomicUnit=on
  Data Store Read : DataStoreRead  DataStoreName=IplusMinv_gyr
  Data Store Read1 : DataStoreRead  DataStoreName=dw
  Data Store Read2 : DataStoreRead  DataStoreName=IplusMinv_acc
  Data Store Read3 : DataStoreRead  DataStoreName=df
  Data Store Read4 : DataStoreRead  DataStoreName=Ggyr
  Logical Operator : Logic  Operator=OR  AllPortsSameDT=off  OutDataTypeStr=boolean
  Mean : dspstat3/Mean  run=on  InputProcessing=Columns as channels (frame based)  reset_popup=None  directionMode=Each column  dimension=1  roiEnable=off  roiType=Rectangles  roiPortion=Entire ROI  roiOutput=Individual statistics for each ROI  roiFlag=off  roundingMode=Floor  overflowMode=off  outputDataTypeStr=Inherit: Same as accumulator  outputMin=[]  outputMax=[]  outputLastDataTypeStr=Inherit: Same as accumulator
  Product : Product  Multiplication=Matrix(*)
  Product1 : Product  Multiplication=Matrix(*)
  Product2 : Product  Multiplication=Matrix(*)
  Saturation : Saturate  LowerLimit=0
  Scope : Scope
  Scope1 : Scope
  Scope5 : Scope
  Sum : Sum  Inputs=|+-
  Sum1 : Sum  Inputs=|+-
  Sum2 : Sum  Inputs=|+-
  detectAccelSaturation : Subsystem  TreatAsAtomicUnit=on
  detectGyroSaturation : Subsystem  TreatAsAtomicUnit=on
  set 0x04 bit : Subsystem  TreatAsAtomicUnit=on
  w_comp : Outport
  f_comp : Outport  Port=2
  DtOut : Outport  Port=3
  wires:
  Data Store Read4/1 -> Product2/1
  Product2/1 -> Sum2/2
  Sum2/1 -> Product/2
  Data Store Read3/1 -> DT police/1(In1), Sum1/2
  f_ib^b/1 -> detectAccelSaturation/1(In1), Sum1/1
  Sum1/1 -> Product1/2
  Data Store Read2/1 -> DT police1/1(In1), Product1/1
  Product1/1 -> Scope1/1, f_comp/1, Product2/2
  Data Store Read/1 -> Product/1
  Sum/1 -> Sum2/1
  w_ib^b/1 -> Sum/1, detectGyroSaturation/1(In1)
  Data Store Read1/1 -> Sum/2
  Dt/1 -> Compare To Constant1/1, Compare To Constant/1, Saturation/1
  Product/1 -> Scope/1, w_comp/1
  Compare To Constant/1 -> Logical Operator/1
  Compare To Constant1/1 -> Logical Operator/2
  Logical Operator/1 -> set 0x04 bit/Enable
  Saturation/1 -> Mean/1, DtOut/1
  Mean/1 -> Scope5/1

== system VINS/setup1 ==

== system VINS/setup2 ==

== system VINS/setup3 ==

== system VINS/stilltimes ==
  note: TODO: If tight still time is exactly zero for 0.1 seconds, reset loose still time to zero.
  w : Inport
  f : Inport  Port=2
  Dt : Inport  Port=3
  Constant : Constant  Value=0.0032
  Constant1 : Constant  Value=0.035
  Constant2 : Constant  Value=0.013 * 3  OutDataTypeStr=Inherit: Inherit via back propagation
  Constant3 : Constant  Value=0.2 * 3  OutDataTypeStr=Inherit: Inherit via back propagation
  DT police : Subsystem  TreatAsAtomicUnit=on
  DT police1 : Subsystem  TreatAsAtomicUnit=on
  Moving Average : dspstat3/Moving Average  Method=Sliding window  ForgettingFactorPort=off  SpecifyWindowLength=on  WindowLength=1000  ForgettingFactor=0.9  SimulateUsing=Code generation
  Mux : Mux  Inputs=2
  Reshape : Reshape  OutputDimensionality=Row vector (2-D)
  Scope6 : Scope
  updateStilltimeLoose : MATLAB Function  TreatAsAtomicUnit=on
  updateStilltimeTight : MATLAB Function  TreatAsAtomicUnit=on
  stilltimes : Outport
  favgs : Outport  Port=2
  wavgs : Outport  Port=3
  wires:
  f/1 -> updateStilltimeTight/2(f), updateStilltimeLoose/2(f)
  Dt/1 -> updateStilltimeTight/3(Dt), updateStilltimeLoose/3(Dt)
  w/1 -> Reshape/1, updateStilltimeTight/1(w), updateStilltimeLoose/1(w)
  Constant/1 -> updateStilltimeTight/4(wsigma)
  Constant1/1 -> updateStilltimeTight/5(fsigma)
  Constant2/1 -> DT police/1(In1), updateStilltimeLoose/4(wsigma)
  Constant3/1 -> DT police1/1(In1), updateStilltimeLoose/5(fsigma)
  updateStilltimeLoose/1(stilltime) -> Mux/2
  updateStilltimeTight/1(stilltime) -> Mux/1
  Mux/1 -> stilltimes/1
  Reshape/1 -> Moving Average/1
  Moving Average/1 -> Scope6/1
  updateStilltimeLoose/2(favgs) -> favgs/1
  updateStilltimeLoose/3(wavgs) -> wavgs/1

== system VINS/timeUpdate ==
  start : Inport
  Dt : Inport  Port=2
  w : Inport  Port=3
  f : Inport  Port=4
  Enable : EnablePort
  Constant : Constant  Commented=on  Value=numStates
  Data Store Read : DataStoreRead  DataStoreName=Pxx
  Data Store Read1 : DataStoreRead  DataStoreName=Cbn
  Data Store Read2 : DataStoreRead  DataStoreName=Pxc
  Data Store Write : DataStoreWrite  DataStoreName=Pxx
  Data Store Write1 : DataStoreWrite  DataStoreName=Pxc
  MATLAB Function1 : MATLAB Function  Commented=on  TreatAsAtomicUnit=on
  MATLAB Function2 : MATLAB Function  Commented=on  TreatAsAtomicUnit=on
  Matrix Multiply : Product  Multiplication=Matrix(*)
  Permute Dimensions : PermuteDimensions
  Product2 : Product  Inputs=3  Multiplication=Matrix(*)
  Sum : Sum  Inputs=|++
  calculatePhi : MATLAB Function  TreatAsAtomicUnit=on
  calculateQ : MATLAB Function  TreatAsAtomicUnit=on
  done : Outport
  wires:
  Product2/1 -> Sum/1  "Phi*P*Phi'"
  calculateQ/1(Q) -> Sum/2
  Constant/1 -> MATLAB Function2/1(numStates)
  f/1 -> calculateQ/2(f_ib), calculatePhi/2(fbod)
  w/1 -> calculateQ/1(omega), calculatePhi/1(omega)
  Data Store Read1/1 -> calculateQ/4(Cbn), calculatePhi/4(Cbn)
  Sum/1 -> Data Store Write/1  "Phi*P*Phi' + Q"
  Permute Dimensions/1 -> Product2/3  "Phi'"
  Data Store Read/1 -> Product2/2
  calculatePhi/1(Phi) -> Matrix Multiply/1, Product2/1, Permute Dimensions/1  "Phi"
  Dt/1 -> calculateQ/3(Dt), calculatePhi/3(Dt)
  start/1 -> done/1  "this is just to enforce block execution order"
  Data Store Read2/1 -> Matrix Multiply/2
  Matrix Multiply/1 -> Data Store Write1/1
